simulink model "Final2018"  (R2016a)
settings: Solver=VariableStepAuto  StartTime=0.0  StopTime=10.0  RelTol=1e-3
values from neighbouring files (symbols this model uses):
  A1 = -A(1,1)    [FInal2019.m]    (also in FInal_3_12_2021.m; Final2017.m; Final2018.m; Final2020feb.m)
  A2 = -A(1,2)    [FInal2019.m]    (also in FInal_3_12_2021.m; Final2017.m; Final2018.m; Final2020feb.m)
  A3 = -A(1,3)    [FInal2019.m]    (also in FInal_3_12_2021.m; Final2017.m; Final2018.m; Final2020feb.m)
  K1 = K(1,1)    [FInal2019.m]    (also in FInal_3_12_2021.m = khat(1,1); Final2017.m; Final2018.m; Final2020feb.m = khat(1,1))
  K2 = K(1,2)    [FInal2019.m]    (also in FInal_3_12_2021.m = khat(1,2); Final2017.m; Final2018.m; Final2020feb.m = khat(1,2))
  K3 = K(1,3)    [FInal2019.m]    (also in FInal_3_12_2021.m = khat(1,3); Final2017.m; Final2018.m; Final2020feb.m = khat(1,3))
settings Model: Creator=alber  LastModifiedBy=alber

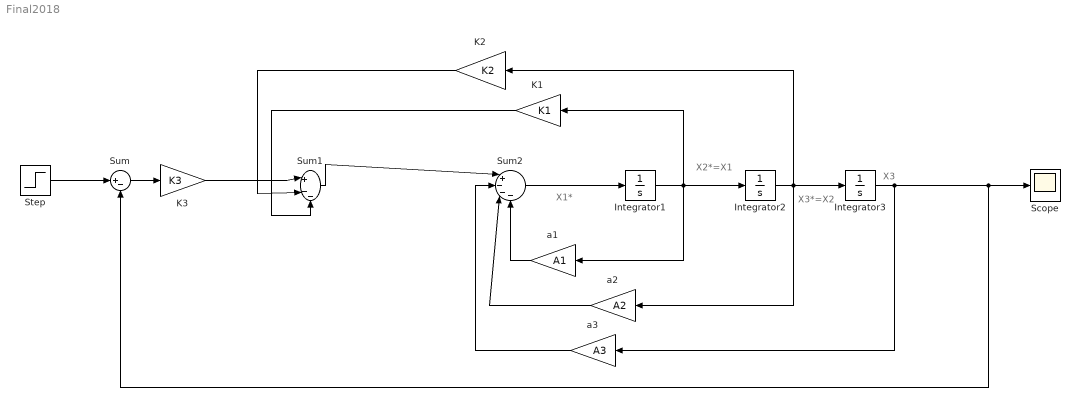
== system Final2018 ==
  note: X3
  note: X3*=X2
  note: X2*=X1
  note: X1*
  Integrator1 : Integrator
  Integrator2 : Integrator
  Integrator3 : Integrator
  K1 : Gain  Gain=K1
  K2 : Gain  Gain=K2
  K3 : Gain  Gain=K3
  Scope : Scope
  Step : Step  SampleTime=0
  Sum : Sum  Inputs=|+-
  Sum1 : Sum  Inputs=|+--
  Sum2 : Sum  Inputs=|+---
  a1 : Gain  Gain=A1
  a2 : Gain  Gain=A2
  a3 : Gain  Gain=A3
  wires:
  Sum/1 -> K3/1
  Sum2/1 -> Integrator1/1
  Integrator1/1 -> K1/1, a1/1, Integrator2/1
  Integrator2/1 -> Integrator3/1, K2/1, a2/1
  Step/1 -> Sum/1
  K1/1 -> Sum1/3
  Sum1/1 -> Sum2/1
  a1/1 -> Sum2/4
  a2/1 -> Sum2/3
  a3/1 -> Sum2/2
  K3/1 -> Sum1/1
  K2/1 -> Sum1/2
  Integrator3/1 -> Scope/1, Sum/2, a3/1
